simulink model "State_space_model"  (R2025b)
settings: Solver=VariableStepAuto  StartTime=0.0  StopTime=20  FixedStep=0.001  RelTol=1e-3
undefined symbols (not defined in the file): den_G, K, Nu, num_G, Nx
settings Model: Creator=Enrico  LastModifiedBy=farin
settings DataIOCC: ReturnWorkspaceOutputsName=out_black_box

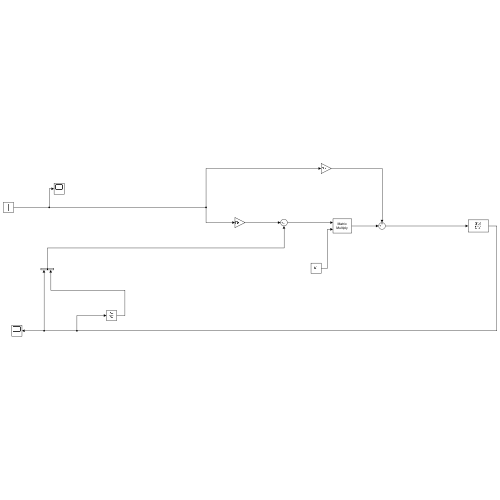
[thumbnail: Simulink's stored preview of the top-level diagram]
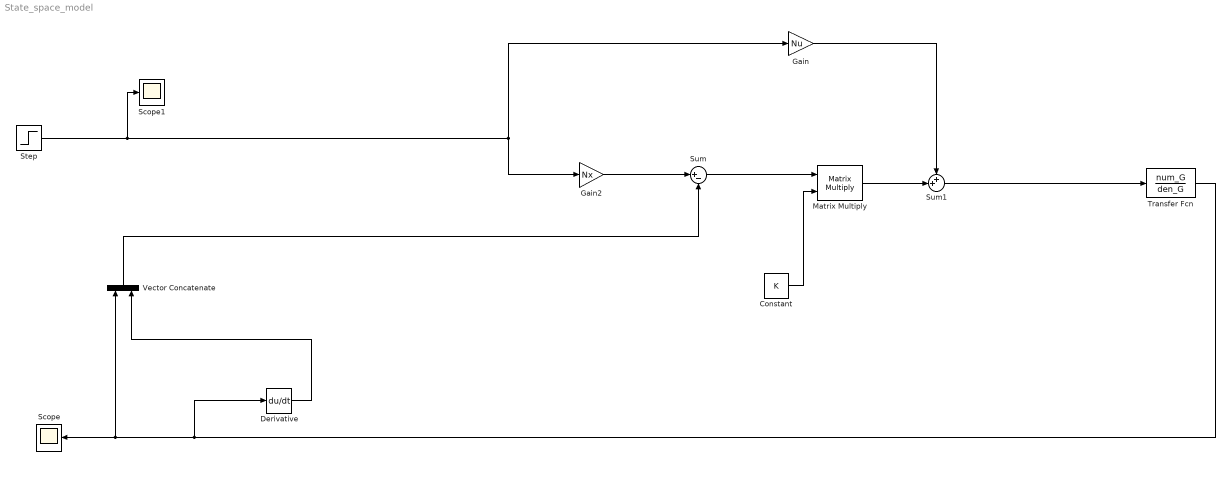
== system State_space_model ==
  Constant : Constant  Value=K
  Derivative : Derivative
  Gain : Gain  Gain=Nu
  Gain2 : Gain  Gain=Nx
  Matrix Multiply : Product  Multiplication=Matrix(*)
  Scope : Scope
      settings: ActiveDisplayYMinimum=0.0024538323374758142  ActiveDisplayYMaximum=0.917535895593973
  Scope1 : Scope
      settings: ActiveDisplayYMinimum=0.10992598764248118  ActiveDisplayYMaximum=1.0893336957280548
  Step : Step  SampleTime=0
  Sum : Sum  Inputs=|+-
  Sum1 : Sum  Inputs=++|
  Transfer Fcn : TransferFcn  Numerator=num_G  Denominator=den_G
  Vector Concatenate : Concatenate
  wires:
  Transfer Fcn/1 -> Derivative/1, Scope/1, Vector Concatenate/1
  Derivative/1 -> Vector Concatenate/2
  Vector Concatenate/1 -> Sum/2
  Step/1 -> Scope1/1, Gain2/1, Gain/1
  Gain/1 -> Sum1/1
  Gain2/1 -> Sum/1
  Sum1/1 -> Transfer Fcn/1
  Sum/1 -> Matrix Multiply/1
  Constant/1 -> Matrix Multiply/2
  Matrix Multiply/1 -> Sum1/2
